simulink model "subsystem"  (Simulink 7.6)
settings: Solver=FixedStepDiscrete  StartTime=0.0  StopTime=1000  RelTol=1e-3
libraries: dsp_blocks x7, simulink x2
settings Model: Creator=Grishma  LastModifiedBy=Joshan
settings DebuggingCC: FcnCallInpInsideContextMsg=Enable All
settings GRTTargetCC: CombineOutputUpdateFcns=on

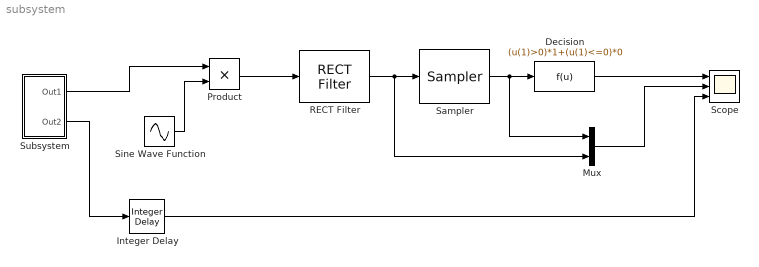
== system subsystem ==
  Decision : Fcn  Expr=(u(1)>0)*1+(u(1)<=0)*0
  Integer Delay : simulink/Discrete/Integer Delay  NumDelays=16  vinit=0.0  samptime=-1
  Mux : Mux  Inputs=2
  Product : Product  RndMeth=Zero
  RECT Filter : dsp_blocks/Filters/RECT Filter  SystemSampleTime=-1  f0=0  f1=0.1  filt_len=32
  Sampler : dsp_blocks/Conversions/Sampler  SystemSampleTime=-1  offset=80  samp_period=50
  Scope : Scope  NumInputPorts=3
      settings: TimeRange=10  YMin=-5~-5~-5  YMax=5~5~5
  Sine Wave Function : Sin  Amplitude=2  Frequency=2*pi*0.1  SampleTime=0
  Subsystem : Subsystem
  wires:
  Subsystem/2(Out2) -> Integer Delay/1
  Sine Wave Function/1 -> Product/2
  Subsystem/1(Out1) -> Product/1
  Product/1 -> RECT Filter/1
  RECT Filter/1 -> Sampler/1, Mux/2
  Sampler/1 -> Decision/1, Mux/1
  Mux/1 -> Scope/2
  Integer Delay/1 -> Scope/3
  Decision/1 -> Scope/1

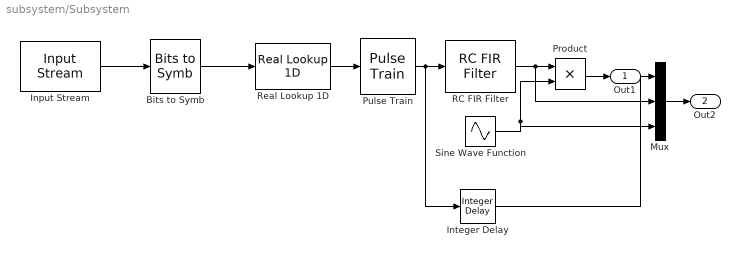
== system subsystem/Subsystem ==
  Bits to Symb : dsp_blocks/Conversions/Bits to Symb  SystemSampleTime=-1
  Input Stream : dsp_blocks/Sources//Sinks/Input Stream  SystemSampleTime=-1  period=10  width=1  fname=rand.mat
  Integer Delay : simulink/Discrete/Integer Delay  NumDelays=16  vinit=0.0  samptime=-1
  Mux : Mux  Inputs=3
  Product : Product  RndMeth=Zero
  Pulse Train : dsp_blocks/Conversions/Pulse Train  SystemSampleTime=-1  period=50
  RC FIR Filter : dsp_blocks/Filters/RC FIR Filter  SystemSampleTime=-1  period=10  beta=0.5  root=off  filt_len=128  win_type=on
  Real Lookup 1D : dsp_blocks/Conversions/Real Lookup 1D  SystemSampleTime=-1  table=[-1 1]
  Sine Wave Function : Sin  Frequency=2*pi*0.1  SampleTime=0
  Out1 : Outport
  Out2 : Outport  Port=2
  wires:
  Bits to Symb/1 -> Real Lookup 1D/1
  Input Stream/1 -> Bits to Symb/1
  Real Lookup 1D/1 -> Pulse Train/1
  Pulse Train/1 -> RC FIR Filter/1, Integer Delay/1
  RC FIR Filter/1 -> Product/1, Mux/2
  Sine Wave Function/1 -> Product/2, Mux/3
  Integer Delay/1 -> Mux/1
  Product/1 -> Out1/1
  Mux/1 -> Out2/1
